simulink model "ModeloBalancin"  (R2024a)
settings: Solver=VariableStepAuto  StartTime=0.0  StopTime=10.0  RelTol=1e-3
undefined symbols (not defined in the file): betaF, g, J, Kf, Lb, Lm, m_b, m_m
settings Model: Creator=Cami  LastModifiedBy=alfar

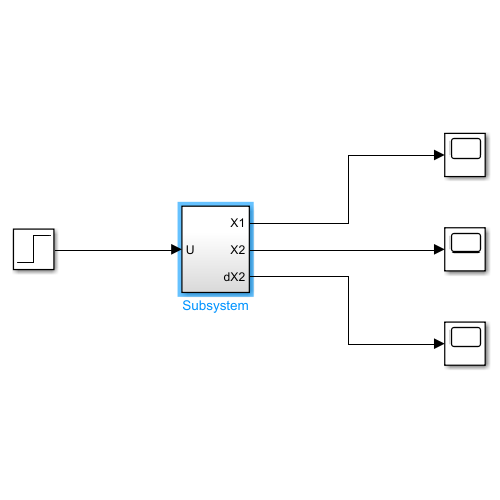
[thumbnail: Simulink's stored preview of the top-level diagram]
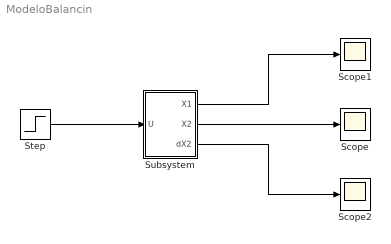
== system ModeloBalancin ==
  Scope : Scope
  Scope1 : Scope
  Scope2 : Scope
  Step : Step  SampleTime=0
  Subsystem : Subsystem
  wires:
  Step/1 -> Subsystem/1(U)
  Subsystem/1(X1) -> Scope1/1
  Subsystem/2(X2) -> Scope/1
  Subsystem/3(dX2) -> Scope2/1

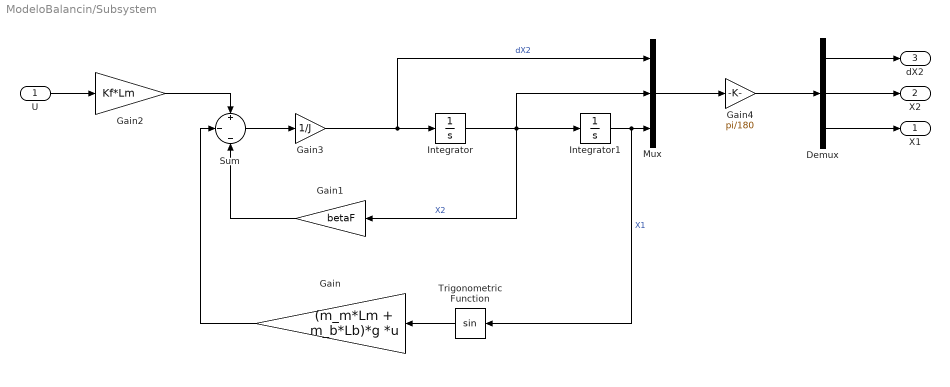
== system ModeloBalancin/Subsystem ==
  U : Inport
  Demux : Demux  Outputs=3
  Gain : Gain  Gain=(m_m*Lm + m_b*Lb)*g  Multiplication=Matrix(K*u)
  Gain1 : Gain  Gain=betaF
  Gain2 : Gain  Gain=Kf*Lm
  Gain3 : Gain  Gain=1/J
  Gain4 : Gain  Gain=pi/180
  Integrator : Integrator
  Integrator1 : Integrator
  Mux : Mux  Inputs=3
  Sum : Sum  Inputs=+|-|-
  Trigonometric Function : Trigonometry
  X1 : Outport
  X2 : Outport  Port=2
  dX2 : Outport  Port=3
  wires:
  Integrator/1 -> Mux/2, Gain1/1, Integrator1/1  "X2"
  Sum/1 -> Gain3/1
  Gain1/1 -> Sum/3
  Demux/3 -> X1/1
  Trigonometric Function/1 -> Gain/1
  Integrator1/1 -> Trigonometric Function/1, Mux/3  "X1"
  Demux/2 -> X2/1
  Gain3/1 -> Mux/1, Integrator/1  "dX2"
  Mux/1 -> Gain4/1
  Gain2/1 -> Sum/1
  Demux/1 -> dX2/1
  Gain/1 -> Sum/2
  Gain4/1 -> Demux/1
  U/1 -> Gain2/1
